simulink model "fft_core"  (Simulink 7.0)
settings: Solver=ode45  StartTime=0.0  StopTime=1  RelTol=1e-3
libraries: xbsIndex_r4 x1118, casper_library x76
(part 12 of 14)

== system fft_core/fft/biplex_core/fft_stage_10/butterfly_direct/twiddle/coeff_gen ==
  rst : Inport
  Counter : xbsIndex_r4/Counter  cnt_type=Free Running  cnt_to=Inf  operation=Up  start_count=0  cnt_by_val=1  arith_type=Unsigned  n_bits=10  bin_pt=0  load_pin=off  rst=on  en=off  explicit_period=on  period=1  dbl_ovrd=off  use_behavioral_HDL=off  use_rpm=off  implementation=Fabric  block_type=counter
      settings: block_version=11.4
  ROM : xbsIndex_r4/ROM  depth=512  initVector="[1                                      0                       0.70709228515625                      -0.70709228515625                       0.92388916015625                       -0.3826904296875                        0.3826904296875                      -0.92388916015625                       0.98077392578125                     -0.195098876953125                      0.555572509765625                      -0.83148193359375                       0.83148193359375                     -0.555572509765625                      0.195098876953125                      -0.98077392578125                       0.99517822265625                       -0.0980224609375                        0.6343994140625                      -0.77301025390625                      0.881927490234375                     -0.471405029296875                         0.290283203125                     -0.956939697265625                      0.956939697265625                        -0.290283203125                      0.471405029296875                     -0.881927490234375                       0.77301025390625                       -0.6343994140625                        0.0980224609375                      -0.99517822265625                      0.998809814453125                        -0.049072265625                       0.67156982421875                     -0.740936279296875                       0.90399169921875                      -0.42755126953125                      0.336883544921875                     -0.941558837890625                       0.97003173828125                      -0.24298095703125                       0.51409912109375                      -0.85772705078125                          0.80322265625                           -0.595703125                         0.146728515625                     -0.989166259765625                      0.989166259765625                        -0.146728515625                            0.595703125                         -0.80322265625                       0.85772705078125                      -0.51409912109375                       0.24298095703125                      -0.97003173828125                      0.941558837890625                     -0.336883544921875                       0.42755126953125                      -0.90399169921875                      0.740936279296875                      -0.67156982421875                         0.049072265625                     -0.998809814453125                       0.99969482421875                       -0.0245361328125                      0.689544677734375                       -0.7242431640625                      0.914215087890625                     -0.405242919921875                      0.359893798828125                       -0.9329833984375                        0.9757080078125                       -0.2191162109375                      0.535003662109375                       -0.8448486328125                      0.817596435546875                       -0.5758056640625                       0.17095947265625                      -0.98529052734375                       0.99249267578125                     -0.122406005859375                            0.615234375                     -0.788360595703125                      0.870086669921875                     -0.492889404296875                        0.2667236328125                     -0.963775634765625                       0.94952392578125                     -0.313690185546875                      0.449615478515625                     -0.893218994140625                        0.7572021484375                     -0.653167724609375                      0.073577880859375                     -0.997283935546875                      0.997283935546875                     -0.073577880859375                      0.653167724609375                       -0.7572021484375                      0.893218994140625                     -0.449615478515625                      0.313690185546875 ...(+15932 chars)]"  distributed_mem=Block RAM  rst=off  init_reg=0  en=off  latency=2  arith_type="Signed  (2's comp)"  n_bits=17  bin_pt=15  dbl_ovrd=off  optimize=Area  use_rpm=on  block_type=sprom
      settings: block_version=11.4
  ROM1 : xbsIndex_r4/ROM  depth=512  initVector="[0                                     -1                      -0.70709228515625                      -0.70709228515625                       -0.3826904296875                      -0.92388916015625                      -0.92388916015625                       -0.3826904296875                     -0.195098876953125                      -0.98077392578125                      -0.83148193359375                     -0.555572509765625                     -0.555572509765625                      -0.83148193359375                      -0.98077392578125                     -0.195098876953125                       -0.0980224609375                      -0.99517822265625                      -0.77301025390625                       -0.6343994140625                     -0.471405029296875                     -0.881927490234375                     -0.956939697265625                        -0.290283203125                        -0.290283203125                     -0.956939697265625                     -0.881927490234375                     -0.471405029296875                       -0.6343994140625                      -0.77301025390625                      -0.99517822265625                       -0.0980224609375                        -0.049072265625                     -0.998809814453125                     -0.740936279296875                      -0.67156982421875                      -0.42755126953125                      -0.90399169921875                     -0.941558837890625                     -0.336883544921875                      -0.24298095703125                      -0.97003173828125                      -0.85772705078125                      -0.51409912109375                           -0.595703125                         -0.80322265625                     -0.989166259765625                        -0.146728515625                        -0.146728515625                     -0.989166259765625                         -0.80322265625                           -0.595703125                      -0.51409912109375                      -0.85772705078125                      -0.97003173828125                      -0.24298095703125                     -0.336883544921875                     -0.941558837890625                      -0.90399169921875                      -0.42755126953125                      -0.67156982421875                     -0.740936279296875                     -0.998809814453125                        -0.049072265625                       -0.0245361328125                      -0.99969482421875                       -0.7242431640625                     -0.689544677734375                     -0.405242919921875                     -0.914215087890625                       -0.9329833984375                     -0.359893798828125                       -0.2191162109375                       -0.9757080078125                       -0.8448486328125                     -0.535003662109375                       -0.5758056640625                     -0.817596435546875                      -0.98529052734375                      -0.17095947265625                     -0.122406005859375                      -0.99249267578125                     -0.788360595703125                           -0.615234375                     -0.492889404296875                     -0.870086669921875                     -0.963775634765625                       -0.2667236328125                     -0.313690185546875                      -0.94952392578125                     -0.893218994140625                     -0.449615478515625                     -0.653167724609375                       -0.7572021484375                     -0.997283935546875                     -0.073577880859375                     -0.073577880859375                     -0.997283935546875                       -0.7572021484375                     -0.653167724609375                     -0.449615478515625                     -0.893218994140625                      -0.94952392578125 ...(+15932 chars)]"  distributed_mem=Block RAM  rst=off  init_reg=0  en=off  latency=2  arith_type="Signed  (2's comp)"  n_bits=17  bin_pt=15  dbl_ovrd=off  optimize=Area  use_rpm=on  block_type=sprom
      settings: block_version=11.4
  Slice : xbsIndex_r4/Slice  nbits=9  boolean_output=off  mode=Upper Bit Location + Width  bit1=0  base1=MSB of Input  bit0=0  base0=LSB of Input  dbl_ovrd=off  block_type=slice
  ri_to_c : casper_library/Misc/ri_to_c  SystemSampleTime=-1
  w : Outport
  wires:
  ri_to_c/1 -> w/1
  rst/1 -> Counter/1
  Counter/1 -> Slice/1
  Slice/1 -> ROM/1, ROM1/1
  ROM/1 -> ri_to_c/1
  ROM1/1 -> ri_to_c/2
